simulink model "TrajectoryFollowDemo"  (Simulink 8.2)
settings: Solver=FixedStepDiscrete  StartTime=0.0  StopTime=Inf  RelTol=1e-3
PreLoadFcn:
  | Ts=0.001;
undefined symbols (not defined in the file or in its folder): DiscIntNeverNeededParam
libraries: simulink x8, xpclib x6, speedgoatlib_IO102 x4, speedgoatlib_IO301 x4, xpcutilitieslib x3
settings Model: Creator=LukePH  LastModifiedBy=LukePH  SimulationMode=external  BufferReuse=off
settings DataIOCC: SignalLoggingSaveFormat=Dataset
settings OptimizationCC: BlockReduction=off  OptimizeBlockIOStorage=off  BufferReuse=off  ExpressionFolding=off  ExpressionDepthLimit=128  LocalBlockOutputs=off
settings DebuggingCC: FcnCallInpInsideContextMsg=EnableAllAsError  StateNameClashWarn=none
settings HardwareCC: ProdIntDivRoundTo=Zero  ProdEndianess=LittleEndian  ProdHWDeviceType=Generic->32-bit x86 compatible
settings RTWCC: SystemTargetFile=xpctarget.tlc  TemplateMakefile=xpc_default_tmf  Description=xPC Target  ProcessScript=xpctarget_make_rtw_hook  RTWCompilerOptimization=On
settings xpcTargetCC: TargetFcnLib=ansi_tfl_table_tmw.mat  CodeReplacementLibrary=XPC_BLAS  ParMdlRefBuildCompliant=on  ConcurrentExecutionCompliant=on  CombineSignalStateStructs=off  MATLABClassNameForMDSCustomization=xpcAperiodicCustomization  GRTInterface=on  GenerateAllocFcn=off  xPCTaskExecutionProfile=off  xPCRL32EventNumber=5000  xPCLoadParamSetFile=off  xPCConcurrentTasks=off  xPCEnableSFAnimation=off

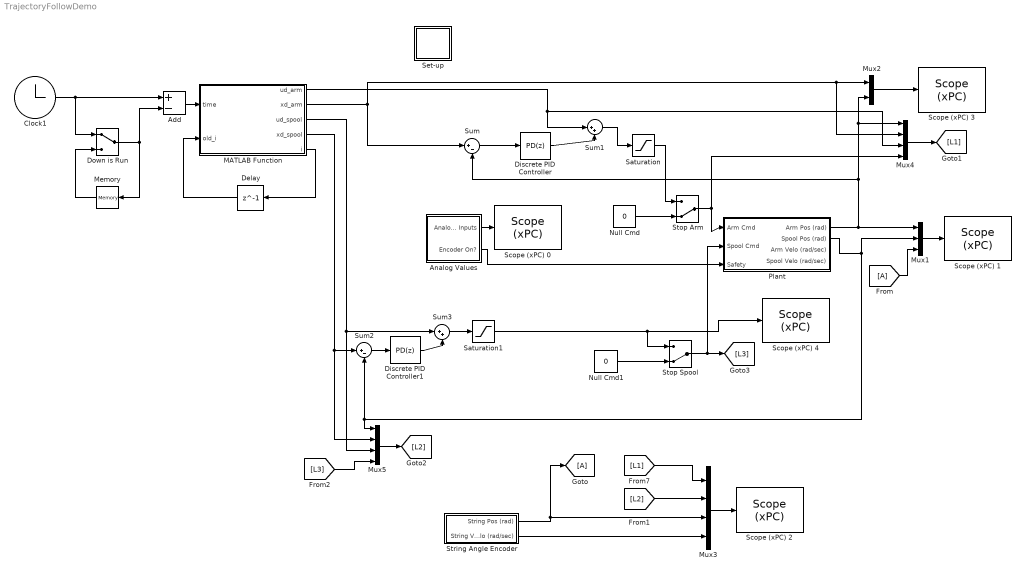
== system TrajectoryFollowDemo ==
  Add : Sum  Inputs=+-
  Analog Values : Subsystem
  Clock1 : Clock
      settings: Decimation=5
  Delay : Delay  DelayLength=1  InitialCondition=1
  Discrete PID Controller : simulink/Continuous/PID Controller  Controller=PD  TimeDomain=Discrete-time  SampleTime=Ts  IntegratorMethod=Forward Euler  FilterMethod=Forward Euler  Form=Parallel  P=30  I=0  D=.15  N=100  InitialConditionSource=internal  InitialConditionForIntegrator=0  InitialConditionForFilter=0  ExternalReset=none  LimitOutput=on  UpperSaturationLimit=6  LowerSaturationLimit=-6  LinearizeAsGain=off  AntiWindupMode=clamping  Kb=1  TrackingMode=off  Kt=1  PParamMin=[]  PParamMax=[]  IParamMin=[]  IParamMax=[]  DParamMin=[]  DParamMax=[]  NParamMin=[]  NParamMax=[]  KbParamMin=[]  KbParamMax=[]  KtParamMin=[]  KtParamMax=[]  POutMin=[]  POutMax=[]  IOutMin=[]  IOutMax=[]  DOutMin=[]  DOutMax=[]  NOutMin=[]  NOutMax=[]  KbOutMin=[]  KbOutMax=[]  KtOutMin=[]  KtOutMax=[]  IntegratorOutMin=[]  IntegratorOutMax=[]  FilterOutMin=[]  FilterOutMax=[]  SumOutMin=[]  SumOutMax=[]  SumI1OutMin=[]  SumI1OutMax=[]  SumI2OutMin=[]  SumI2OutMax=[]  SumI3OutMin=[]  SumI3OutMax=[]  SumDOutMin=[]  SumDOutMax=[]  SaturationOutMin=[]  SaturationOutMax=[]  IntegratorContinuousStateAttributes=''  IntegratorStateMustResolveToSignalObject=off  IntegratorRTWStateStorageClass=Auto  FilterContinuousStateAttributes=''  FilterStateMustResolveToSignalObject=off  FilterRTWStateStorageClass=Auto
  Discrete PID Controller1 : simulink/Continuous/PID Controller  Controller=PD  TimeDomain=Discrete-time  SampleTime=Ts  IntegratorMethod=Forward Euler  FilterMethod=Forward Euler  Form=Parallel  P=20  I=0  D=.05  N=100  InitialConditionSource=internal  InitialConditionForIntegrator=0  InitialConditionForFilter=0  ExternalReset=none  LimitOutput=on  UpperSaturationLimit=6  LowerSaturationLimit=-6  LinearizeAsGain=off  AntiWindupMode=clamping  Kb=1  TrackingMode=off  Kt=1  PParamMin=[]  PParamMax=[]  IParamMin=[]  IParamMax=[]  DParamMin=[]  DParamMax=[]  NParamMin=[]  NParamMax=[]  KbParamMin=[]  KbParamMax=[]  KtParamMin=[]  KtParamMax=[]  POutMin=[]  POutMax=[]  IOutMin=[]  IOutMax=[]  DOutMin=[]  DOutMax=[]  NOutMin=[]  NOutMax=[]  KbOutMin=[]  KbOutMax=[]  KtOutMin=[]  KtOutMax=[]  IntegratorOutMin=[]  IntegratorOutMax=[]  FilterOutMin=[]  FilterOutMax=[]  SumOutMin=[]  SumOutMax=[]  SumI1OutMin=[]  SumI1OutMax=[]  SumI2OutMin=[]  SumI2OutMax=[]  SumI3OutMin=[]  SumI3OutMax=[]  SumDOutMin=[]  SumDOutMax=[]  SaturationOutMin=[]  SaturationOutMax=[]  IntegratorContinuousStateAttributes=''  IntegratorStateMustResolveToSignalObject=off  IntegratorRTWStateStorageClass=Auto  FilterContinuousStateAttributes=''  FilterStateMustResolveToSignalObject=off  FilterRTWStateStorageClass=Auto
  Down is Run : ManualSwitch
  MATLAB Function : MATLAB Function  TreatAsAtomicUnit=on
  Memory : Memory  InheritSampleTime=on
  Mux1 : Mux  Inputs=3
  Mux2 : Mux  Inputs=2
  Mux3 : Mux
  Mux4 : Mux
  Mux5 : Mux
  Null Cmd : Constant  Value=0
  Null Cmd1 : Constant  Value=0
  Plant : Subsystem
  Saturation : Saturate  UpperLimit=6  LowerLimit=-6
  Saturation1 : Saturate  UpperLimit=6  LowerLimit=-6
  "Scope (xPC) 0 " : xpclib/Misc./Scope (xPC)   scopeno=5  scopetype=Target  autostart=on  viewmode=Numerical  formatstr='%15.6f'  grid=on  ylimits=[0,0]  nosamples=250  noprepostsamples=0  interleave=1  triggermode=FreeRun  triggersignal=1  trigsignalfromport=off  triggerlevel=0.0  triggerslope=Either  triggerscope=1  triggersample=0  filename=data.dat  mode=Lazy  writesize=512  autorestart=off  dynamicfilemode=off  maxwritefilesize=512*1024^2
  Scope (xPC) 1 : xpclib/Misc./Scope (xPC)   scopeno=1  scopetype=Target  autostart=on  viewmode=Numerical  formatstr='%15.6f'  grid=on  ylimits=[-2*pi,2*pi]  nosamples=250  noprepostsamples=0  interleave=1  triggermode=FreeRun  triggersignal=1  trigsignalfromport=off  triggerlevel=0.0  triggerslope=Either  triggerscope=1  triggersample=0  filename=data.dat  mode=Lazy  writesize=512  autorestart=off  dynamicfilemode=off  maxwritefilesize=512*1024^2
  Scope (xPC) 2 : xpclib/Misc./Scope (xPC)   scopeno=10  scopetype=File  autostart=on  viewmode=Numerical  formatstr='%15.6f'  grid=on  ylimits=[-2*pi,2*pi]  nosamples=4001  noprepostsamples=0  interleave=4  triggermode=FreeRun  triggersignal=1  trigsignalfromport=off  triggerlevel=0.0  triggerslope=Either  triggerscope=1  triggersample=0  filename=data.dat  mode=Lazy  writesize=512  autorestart=on  dynamicfilemode=off  maxwritefilesize=512*1024^2
  Scope (xPC) 3 : xpclib/Misc./Scope (xPC)   scopeno=6  scopetype=Target  autostart=on  viewmode=Graphical redraw  formatstr='%15.6f'  grid=on  ylimits=[-2*pi,2*pi]  nosamples=250  noprepostsamples=0  interleave=1  triggermode=FreeRun  triggersignal=1  trigsignalfromport=off  triggerlevel=0.0  triggerslope=Either  triggerscope=1  triggersample=0  filename=data.dat  mode=Lazy  writesize=512  autorestart=off  dynamicfilemode=off  maxwritefilesize=512*1024^2
  Scope (xPC) 4 : xpclib/Misc./Scope (xPC)   scopeno=3  scopetype=Target  autostart=on  viewmode=Graphical redraw  formatstr='%15.6f'  grid=on  ylimits=[-2*pi,2*pi]  nosamples=250  noprepostsamples=0  interleave=1  triggermode=FreeRun  triggersignal=1  trigsignalfromport=off  triggerlevel=0.0  triggerslope=Either  triggerscope=1  triggersample=0  filename=data.dat  mode=Lazy  writesize=512  autorestart=off  dynamicfilemode=off  maxwritefilesize=512*1024^2
  Set-up : Subsystem
  Stop Arm : ManualSwitch  CurrentSetting=0
  Stop Spool : ManualSwitch  CurrentSetting=0
  String Angle Encoder : Subsystem
  Sum : Sum  Inputs=|+-
  Sum1 : Sum  Inputs=|++
  Sum2 : Sum  Inputs=|+-
  Sum3 : Sum  Inputs=|++
  wires:
  Delay/1 -> MATLAB Function/2(old_i)
  MATLAB Function/5(i) -> Delay/1
  Clock1/1 -> Add/1, Down is Run/1
  Down is Run/1 -> Memory/1, Add/2
  Memory/1 -> Down is Run/2
  Add/1 -> MATLAB Function/1(time)
  Mux2/1 -> Scope (xPC) 3/1
  Analog Values/1(Analog Inputs) -> "Scope (xPC) 0 "/1
  Plant/1(Arm Pos (rad)) -> Mux1/1, Sum/2, Mux2/2, Mux4/1
  Plant/2(Spool Pos (rad)) -> Mux5/1, Sum2/2, Mux1/2
  Analog Values/2(Encoder On?) -> Plant/3(Safety)
  Sum/1 -> Discrete PID Controller/1
  Null Cmd/1 -> Stop Arm/2
  Saturation/1 -> Stop Arm/1
  Stop Arm/1 -> Plant/1(Arm Cmd), Mux4/4
  Stop Spool/1 -> Plant/2(Spool Cmd), [L3]
  Null Cmd1/1 -> Stop Spool/2
  [A] -> Mux1/3
  Mux1/1 -> Scope (xPC) 1/1
  MATLAB Function/2(xd_arm) -> Sum/1, Mux4/2, Mux2/1
  Mux3/1 -> Scope (xPC) 2/1
  String Angle Encoder/1(String Pos (rad)) -> Mux3/3, [A]
  [L2] -> Mux3/2
  [L1] -> Mux3/1
  Discrete PID Controller/1 -> Sum1/2
  Sum1/1 -> Saturation/1
  Sum2/1 -> Discrete PID Controller1/1
  Discrete PID Controller1/1 -> Sum3/2
  Sum3/1 -> Saturation1/1
  MATLAB Function/4(xd_spool) -> Mux5/2, Sum2/1
  MATLAB Function/3(ud_spool) -> Mux5/3, Sum3/1
  MATLAB Function/1(ud_arm) -> Mux4/3, Sum1/1
  Mux4/1 -> [L1]
  Mux5/1 -> [L2]
  [L3] -> Mux5/4
  String Angle Encoder/2(String Velo (rad/sec)) -> Mux3/4
  Saturation1/1 -> Scope (xPC) 4/1, Stop Spool/1

== system TrajectoryFollowDemo/Analog Values ==
  Analog input : speedgoatlib_IO102/Analog input  id=1  channels=[1,2,3,4]  range=1  high_voltage=off  adCoupling=2  ts=Ts  pciSlot=-1
  Constant : Constant  Value=3.25
  Mux : Mux
  Relational Operator : RelationalOperator  Operator=>  OutDataTypeStr=fixdt(1,16)
  Analog Inputs : Outport
  Encoder On? : Outport  Port=2
  wires:
  Mux/1 -> Analog Inputs/1
  Relational Operator/1 -> Encoder On?/1
  Constant/1 -> Relational Operator/2
  Analog input/1 -> Mux/1
  Analog input/2 -> Mux/2
  Analog input/3 -> Mux/3
  Analog input/4 -> Relational Operator/1, Mux/4

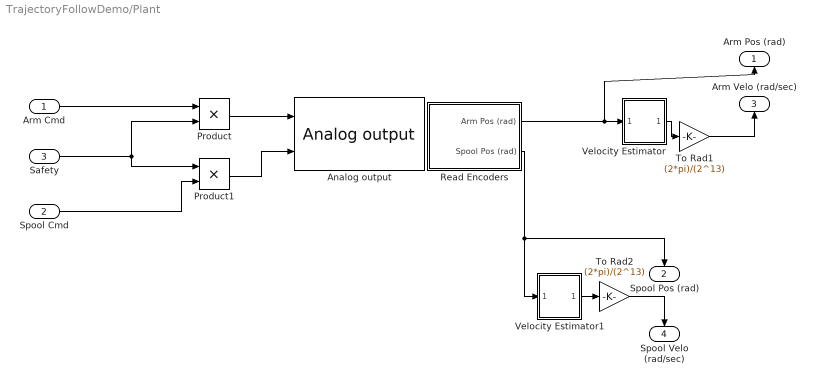
== system TrajectoryFollowDemo/Plant ==
  Arm Cmd : Inport
  Spool Cmd : Inport  Port=2
  Safety : Inport  Port=3
  Analog output : speedgoatlib_IO102/Analog output  id=1  channels=[1,2]  range=1  ts=Ts  pciSlot=-1
  Product : Product
  Product1 : Product
  Read Encoders : Subsystem
  To Rad1 : Gain  Gain=(2*pi)/(2^13)  OutDataTypeStr=double
  To Rad2 : Gain  Gain=(2*pi)/(2^13)  OutDataTypeStr=double
  Velocity Estimator : Subsystem  mask{SampleTime=Ts}
      mask prompts: SampleTime "Sample time (-1 for inherited):"
      mask help:
      | This Block takes in encoder values at a rate of 1 sample per Ts seconds and
      | produces an estimate of the velocity at the given time.
      mask TypeOptions SampleTime: Velocity /SystemSampleTime | Weight Calc/SystemSampleTime | Weighted Average/SystemSampleTime | Velocity /Time Constant/Value | Discrete-Time Integrator/SampleTime | Dead Zone/SampleTime | Weight Calc/9000 rad//sec^2 Cut-off/SampleTime | Weight Calc/Discrete Low Pass1/SampleTime | Weight Calc/Discrete Transfer Fcn/SampleTime | Weight Calc/Discrete Transfer Fcn1/SampleTime | Discrete Low Pass2/SampleTime | Velocity /My Difference/Delay/SampleTime | Velocity /My Difference/Sum/SampleTime
      mask Display:
      | port_label('output', 1, '')
      | port_label('input', 1, '')
  Velocity Estimator1 : Subsystem  mask{SampleTime=Ts}
      mask prompts: SampleTime "Sample time (-1 for inherited):"
      mask help:
      | This Block takes in encoder values at a rate of 1 sample per Ts seconds and
      | produces an estimate of the velocity at the given time.
      mask TypeOptions SampleTime: Velocity /SystemSampleTime | Weight Calc/SystemSampleTime | Weighted Average/SystemSampleTime | Velocity /Time Constant/Value | Discrete-Time Integrator/SampleTime | Dead Zone/SampleTime | Weight Calc/9000 rad//sec^2 Cut-off/SampleTime | Weight Calc/Discrete Low Pass1/SampleTime | Weight Calc/Discrete Transfer Fcn/SampleTime | Weight Calc/Discrete Transfer Fcn1/SampleTime | Discrete Low Pass2/SampleTime | Velocity /My Difference/Delay/SampleTime | Velocity /My Difference/Sum/SampleTime
      mask Display:
      | port_label('output', 1, '')
      | port_label('input', 1, '')
  Arm Pos (rad) : Outport
  Spool Pos (rad) : Outport  Port=2
  Arm Velo (rad/sec) : Outport  Port=3
  Spool Velo (rad/sec) : Outport  Port=4
  wires:
  Read Encoders/2(Spool Pos (rad)) -> Velocity Estimator1/1(In1), Spool Pos (rad)/1
  Spool Cmd/1 -> Product1/2
  Product1/1 -> Analog output/2
  Safety/1 -> Product1/1, Product/2
  Read Encoders/1(Arm Pos (rad)) -> Arm Pos (rad)/1, Velocity Estimator/1(In1)
  Arm Cmd/1 -> Product/1
  Product/1 -> Analog output/1
  Velocity Estimator/1(Out1) -> To Rad1/1
  To Rad1/1 -> Arm Velo (rad/sec)/1
  Velocity Estimator1/1(Out1) -> To Rad2/1
  To Rad2/1 -> Spool Velo (rad/sec)/1

== system TrajectoryFollowDemo/Set-up ==
  AnalogSetUp : Subsystem
  Digital output : speedgoatlib_IO301/DIO/Digital output  id=1  channelGroup=Lower  portType=32 ports of type double  lowerDirection=[0,0,0,0,0,0,1,1,1,1,1,1,1,1,1,1]  upperDirection=[1,1,1,1,1,1,1,1,0,0,0,0,0,0,0,0]  ts=Ts  pciSlot=-1
  Disable NST : Constant  Value=0
  Do Not Zero Arm : Constant
  Do Not Zero Spool : Constant
  Setup : speedgoatlib_IO301/Setup/Setup  group=Lower channel group setup  id=1  fpga1=speedgoat_IO301_CI_01230  pciSlot=-1  lowerDirection=[0,0,0,0,0,0,1,1,1,1,1,1,1,1,1,1]  lowerReset=[1]  lowerValue=[1]  upperDirection=[1, 1, 1, 1, 1, 1, 1, 1, 0, 0, 0, 0, 0, 0, 0, 0]  upperReset=[1]  upperValue=[0]
  wires:
  Disable NST/1 -> Digital output/19, Digital output/17
  Do Not Zero Arm/1 -> Digital output/18
  Do Not Zero Spool/1 -> Digital output/20

== system TrajectoryFollowDemo/String Angle Encoder ==
  EncoderPos3 : xpcutilitieslib/Bit Packing   MaskBitPatterns={[0:12]}  MaskPackDataType=int32  MaskPackDataSize=[1]
  SSIM : speedgoatlib_IO301/SSI/SSIM  id=1  chan=[3]  coding=Binary  clockDivider=[200]  wordSize=[13]  TL=[0]  TP=[990]  ssiminv=off  ts=Ts  pciSlot=-1
  To Rad1 : Gain  Gain=(2*pi)/(2^13)  OutDataTypeStr=double
  To Rad4 : Gain  Gain=(2*pi)/(2^13)  OutDataTypeStr=double
  Velocity Estimator : Subsystem  mask{SampleTime=Ts}
      mask prompts: SampleTime "Sample time (-1 for inherited):"
      mask help:
      | This Block takes in encoder values at a rate of 1 sample per Ts seconds and
      | produces an estimate of the velocity at the given time.
      mask TypeOptions SampleTime: Velocity /SystemSampleTime | Weight Calc/SystemSampleTime | Weighted Average/SystemSampleTime | Velocity /Time Constant/Value | Discrete-Time Integrator/SampleTime | Dead Zone/SampleTime | Weight Calc/9000 rad//sec^2 Cut-off/SampleTime | Weight Calc/Discrete Low Pass1/SampleTime | Weight Calc/Discrete Transfer Fcn/SampleTime | Weight Calc/Discrete Transfer Fcn1/SampleTime | Discrete Low Pass2/SampleTime | Velocity /My Difference/Delay/SampleTime | Velocity /My Difference/Sum/SampleTime
      mask Display:
      | port_label('output', 1, '')
      | port_label('input', 1, '')
  String Pos (rad) : Outport
  String Velo (rad/sec) : Outport  Port=2
  wires:
  To Rad4/1 -> String Pos (rad)/1
  SSIM/1 -> EncoderPos3/1
  EncoderPos3/1 -> Velocity Estimator/1(In1), To Rad4/1
  Velocity Estimator/1(Out1) -> To Rad1/1
  To Rad1/1 -> String Velo (rad/sec)/1

== system TrajectoryFollowDemo/Plant/Read Encoders ==
  EncoderPos : xpcutilitieslib/Bit Packing   MaskBitPatterns={[0:16]}  MaskPackDataType=int32  MaskPackDataSize=[1]
  EncoderPos1 : xpcutilitieslib/Bit Packing   MaskBitPatterns={[0:16]}  MaskPackDataType=int32  MaskPackDataSize=[1]
  SSIM : speedgoatlib_IO301/SSI/SSIM  id=1  chan=[1:2]  coding=Gray  clockDivider=[200]  wordSize=[17]  TL=[0]  TP=[990]  ssiminv=off  ts=Ts  pciSlot=-1
  Spike Removal : Subsystem
  To Rad : Gain  Gain=(2*pi)/(2^17)  OutDataTypeStr=double
  To Rad1 : Gain  Gain=-(2*pi)/(2^17)  OutDataTypeStr=double
  Wrap Encoder Values : Subsystem
  Arm Pos (rad) : Outport
  Spool Pos (rad) : Outport  Port=2
  wires:
  SSIM/1 -> EncoderPos/1
  EncoderPos/1 -> To Rad/1
  To Rad/1 -> Arm Pos (rad)/1
  SSIM/2 -> EncoderPos1/1
  To Rad1/1 -> Spool Pos (rad)/1
  Spike Removal/1(Filtered) -> To Rad1/1
  EncoderPos1/1 -> Wrap Encoder Values/1(Raw Input)
  Wrap Encoder Values/1(Wrapped Values) -> Spike Removal/1(Encoder)

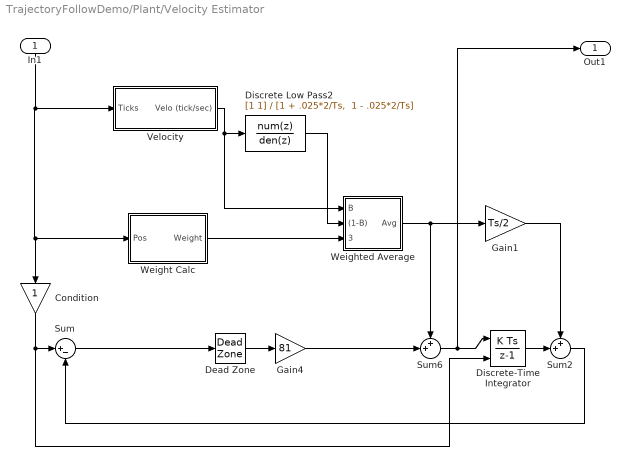
== system TrajectoryFollowDemo/Plant/Velocity Estimator ==
  In1 : Inport
  Condition : Gain  OutMin=0  OutMax=10^9  OutDataTypeStr=double
  Dead Zone : DeadZone  LowerValue=-1  UpperValue=1  SampleTime=SampleTime  SaturateOnIntegerOverflow=on
  Discrete Low Pass2 : DiscreteTransferFcn  Numerator=[1 1]  Denominator="[1 + .025*2/Ts,  1 - .025*2/Ts]"  SampleTime=SampleTime
  Discrete-Time Integrator : DiscreteIntegrator  InitialConditionSource=external  SampleTime=SampleTime  ICPrevOutput=DiscIntNeverNeededParam  ICPrevScaledInput=DiscIntNeverNeededParam
  Gain1 : Gain  Gain=Ts/2
  Gain4 : Gain  Gain=81
  Sum : Sum  Inputs=|+-
  Sum2 : Sum  Inputs=++|
  Sum6 : Sum  Inputs=++|
  "Velocity " : Subsystem  SystemSampleTime=SampleTime
  Weight Calc : Subsystem  SystemSampleTime=SampleTime
  Weighted Average : Subsystem  SystemSampleTime=SampleTime
  Out1 : Outport
  wires:
  Weight Calc/1(Weight) -> Weighted Average/3(Weight)
  Gain1/1 -> Sum2/1
  Discrete-Time Integrator/1 -> Sum2/2
  Sum2/1 -> Sum/2
  Discrete Low Pass2/1 -> Weighted Average/2((1-B))
  Sum6/1 -> Out1/1, Discrete-Time Integrator/1
  Dead Zone/1 -> Gain4/1
  Weighted Average/1(Avg) -> Sum6/1, Gain1/1
  Gain4/1 -> Sum6/2
  Sum/1 -> Dead Zone/1
  "Velocity "/1(Velo (tick/sec)) -> Weighted Average/1("B "), Discrete Low Pass2/1
  In1/1 -> Condition/1, Weight Calc/1(Pos), "Velocity "/1(Ticks)
  Condition/1 -> Discrete-Time Integrator/2, Sum/1

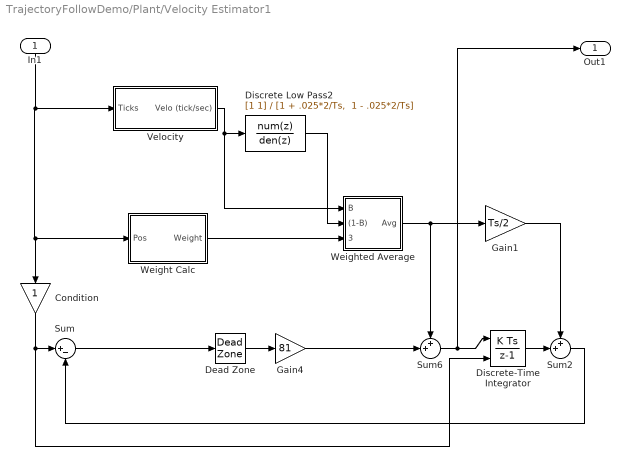
== system TrajectoryFollowDemo/Plant/Velocity Estimator1 ==
  In1 : Inport
  Condition : Gain  OutMin=0  OutMax=10^9  OutDataTypeStr=double
  Dead Zone : DeadZone  LowerValue=-1  UpperValue=1  SampleTime=SampleTime  SaturateOnIntegerOverflow=on
  Discrete Low Pass2 : DiscreteTransferFcn  Numerator=[1 1]  Denominator="[1 + .025*2/Ts,  1 - .025*2/Ts]"  SampleTime=SampleTime
  Discrete-Time Integrator : DiscreteIntegrator  InitialConditionSource=external  SampleTime=SampleTime  ICPrevOutput=DiscIntNeverNeededParam  ICPrevScaledInput=DiscIntNeverNeededParam
  Gain1 : Gain  Gain=Ts/2
  Gain4 : Gain  Gain=81
  Sum : Sum  Inputs=|+-
  Sum2 : Sum  Inputs=++|
  Sum6 : Sum  Inputs=++|
  "Velocity " : Subsystem  SystemSampleTime=SampleTime
  Weight Calc : Subsystem  SystemSampleTime=SampleTime
  Weighted Average : Subsystem  SystemSampleTime=SampleTime
  Out1 : Outport
  wires:
  Weight Calc/1(Weight) -> Weighted Average/3(Weight)
  Gain1/1 -> Sum2/1
  Discrete-Time Integrator/1 -> Sum2/2
  Sum2/1 -> Sum/2
  Discrete Low Pass2/1 -> Weighted Average/2((1-B))
  Sum6/1 -> Out1/1, Discrete-Time Integrator/1
  Dead Zone/1 -> Gain4/1
  Weighted Average/1(Avg) -> Sum6/1, Gain1/1
  Gain4/1 -> Sum6/2
  Sum/1 -> Dead Zone/1
  "Velocity "/1(Velo (tick/sec)) -> Weighted Average/1("B "), Discrete Low Pass2/1
  In1/1 -> Condition/1, Weight Calc/1(Pos), "Velocity "/1(Ticks)
  Condition/1 -> Discrete-Time Integrator/2, Sum/1

== system TrajectoryFollowDemo/Set-up/AnalogSetUp ==
  Analog input : speedgoatlib_IO102/Analog input  Commented=on  id=1  channels=[1,2]  range=1  high_voltage=off  adCoupling=1  ts=Ts  pciSlot=-1
  Mux : Mux  Commented=on  Inputs=2
  Scope (xPC) 1 : xpclib/Misc./Scope (xPC)   Commented=on  scopeno=4  scopetype=Target  autostart=on  viewmode=Graphical redraw  formatstr='%15.6f'  grid=on  ylimits=[0,0]  nosamples=250  noprepostsamples=0  interleave=1  triggermode=FreeRun  triggersignal=1  trigsignalfromport=off  triggerlevel=0.0  triggerslope=Either  triggerscope=1  triggersample=0  filename=data.dat  mode=Lazy  writesize=512  autorestart=off  dynamicfilemode=off  maxwritefilesize=512*1024^2
  SetupAnalog : speedgoatlib_IO102/Setup  group=Analog input setup  id=1  range=+-10V  cal=off  pciSlot=-1  adChannelMode=Multiple-channel (enter number of channels below)  adChannel=4  adCoupling=Single-ended  daChannel=[1,2]  daReset=[1,1]  daInitValue=[0,0]  diChannel=[1]  doChannel=[1]  doReset=[1]  doInitValue=[0]
  wires:
  Mux/1 -> Scope (xPC) 1/1
  Analog input/1 -> Mux/1
  Analog input/2 -> Mux/2

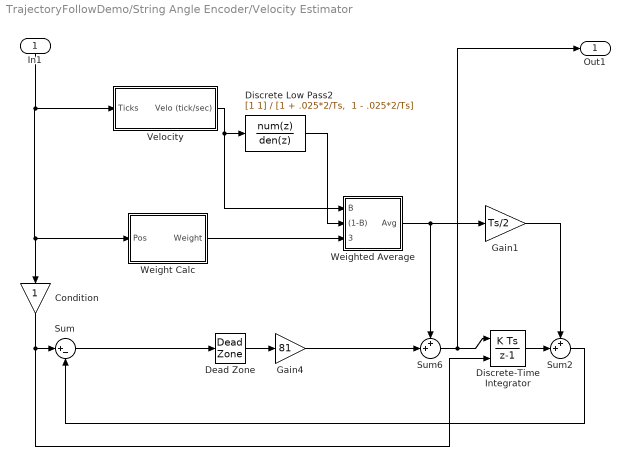
== system TrajectoryFollowDemo/String Angle Encoder/Velocity Estimator ==
  In1 : Inport
  Condition : Gain  OutMin=0  OutMax=10^9  OutDataTypeStr=double
  Dead Zone : DeadZone  LowerValue=-1  UpperValue=1  SampleTime=SampleTime  SaturateOnIntegerOverflow=on
  Discrete Low Pass2 : DiscreteTransferFcn  Numerator=[1 1]  Denominator="[1 + .025*2/Ts,  1 - .025*2/Ts]"  SampleTime=SampleTime
  Discrete-Time Integrator : DiscreteIntegrator  InitialConditionSource=external  SampleTime=SampleTime  ICPrevOutput=DiscIntNeverNeededParam  ICPrevScaledInput=DiscIntNeverNeededParam
  Gain1 : Gain  Gain=Ts/2
  Gain4 : Gain  Gain=81
  Sum : Sum  Inputs=|+-
  Sum2 : Sum  Inputs=++|
  Sum6 : Sum  Inputs=++|
  "Velocity " : Subsystem  SystemSampleTime=SampleTime
  Weight Calc : Subsystem  SystemSampleTime=SampleTime
  Weighted Average : Subsystem  SystemSampleTime=SampleTime
  Out1 : Outport
  wires:
  Weight Calc/1(Weight) -> Weighted Average/3(Weight)
  Gain1/1 -> Sum2/1
  Discrete-Time Integrator/1 -> Sum2/2
  Sum2/1 -> Sum/2
  Discrete Low Pass2/1 -> Weighted Average/2((1-B))
  Sum6/1 -> Out1/1, Discrete-Time Integrator/1
  Dead Zone/1 -> Gain4/1
  Weighted Average/1(Avg) -> Sum6/1, Gain1/1
  Gain4/1 -> Sum6/2
  Sum/1 -> Dead Zone/1
  "Velocity "/1(Velo (tick/sec)) -> Weighted Average/1("B "), Discrete Low Pass2/1
  In1/1 -> Condition/1, Weight Calc/1(Pos), "Velocity "/1(Ticks)
  Condition/1 -> Discrete-Time Integrator/2, Sum/1

== system TrajectoryFollowDemo/Plant/Read Encoders/Spike Removal ==
  Encoder : Inport
  Abs1 : Abs
  Delay1 : Delay  DelayLength=1  InitialCondition=0  SampleTime=Ts
  Memory1 : Memory  InheritSampleTime=on
  Relational Operator2 : RelationalOperator  OutDataTypeStr=boolean
  Spike height : Constant  Value=130000
  Sum2 : Sum  Inputs=|-+
  Switch2 : Switch  Criteria=u2 > Threshold  SampleTime=Ts
  Filtered : Outport
  wires:
  Switch2/1 -> Filtered/1, Memory1/1
  Delay1/1 -> Sum2/1
  Memory1/1 -> Switch2/1
  Encoder/1 -> Sum2/2, Switch2/3, Delay1/1
  Abs1/1 -> Relational Operator2/1
  Spike height/1 -> Relational Operator2/2
  Sum2/1 -> Abs1/1
  Relational Operator2/1 -> Switch2/2

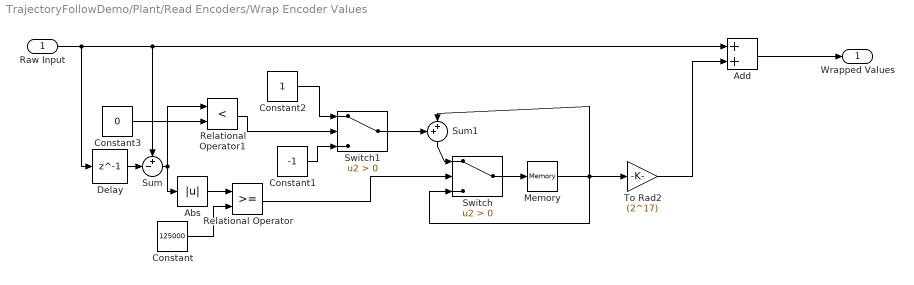
== system TrajectoryFollowDemo/Plant/Read Encoders/Wrap Encoder Values ==
  Raw Input : Inport
  Abs : Abs
  Add : Sum
  Constant : Constant  Value=125000
  Constant1 : Constant  Value=-1
  Constant2 : Constant
  Constant3 : Constant  Value=0
  Delay : Delay  DelayLength=1  InitialCondition=0  SampleTime=Ts
  Memory : Memory  InheritSampleTime=on
  Relational Operator : RelationalOperator  OutDataTypeStr=boolean
  Relational Operator1 : RelationalOperator  Operator=<  OutDataTypeStr=boolean
  Sum : Sum  Inputs=+-|
  Sum1 : Sum  Inputs=++|
  Switch : Switch  Criteria=u2 > Threshold  SampleTime=Ts
  Switch1 : Switch  Criteria=u2 > Threshold  SampleTime=Ts
  To Rad2 : Gain  Gain=(2^17)  OutDataTypeStr=double
  Wrapped Values : Outport
  wires:
  Raw Input/1 -> Delay/1, Sum/1, Add/1
  Add/1 -> Wrapped Values/1
  Constant/1 -> Relational Operator/2
  Relational Operator/1 -> Switch/2
  Sum1/1 -> Switch/1
  Delay/1 -> Sum/2
  Switch/1 -> Memory/1
  Memory/1 -> Sum1/2, Switch/3, To Rad2/1
  Switch1/1 -> Sum1/1
  Constant1/1 -> Switch1/3
  Relational Operator1/1 -> Switch1/2
  Constant2/1 -> Switch1/1
  Sum/1 -> Relational Operator1/1, Abs/1
  Abs/1 -> Relational Operator/1
  Constant3/1 -> Relational Operator1/2
  To Rad2/1 -> Add/2

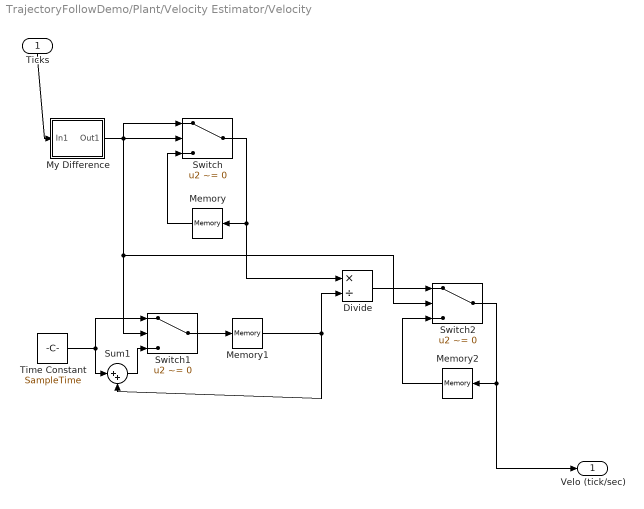
== system TrajectoryFollowDemo/Plant/Velocity Estimator/Velocity  ==
  Ticks : Inport  SampleTime=Ts
  Divide : Product  Inputs=*/
  Memory : Memory
  Memory1 : Memory  X0=Ts
  Memory2 : Memory
  My Difference : Subsystem
  Sum1 : Sum  Inputs=|++
  Switch : Switch  Criteria=u2 ~= 0
  Switch1 : Switch  Criteria=u2 ~= 0
  Switch2 : Switch  Criteria=u2 ~= 0
  Time Constant : Constant  Value=SampleTime
  Velo (tick/sec) : Outport  SampleTime=Ts
  wires:
  Ticks/1 -> My Difference/1(In1)
  My Difference/1(Out1) -> Switch/1, Switch1/2, Switch2/2, Switch/2
  Switch/1 -> Divide/1, Memory/1
  Memory/1 -> Switch/3
  Switch1/1 -> Memory1/1
  Time Constant/1 -> Switch1/1, Sum1/1
  Sum1/1 -> Switch1/3
  Memory1/1 -> Sum1/2, Divide/2
  Divide/1 -> Switch2/1
  Memory2/1 -> Switch2/3
  Switch2/1 -> Velo (tick/sec)/1, Memory2/1

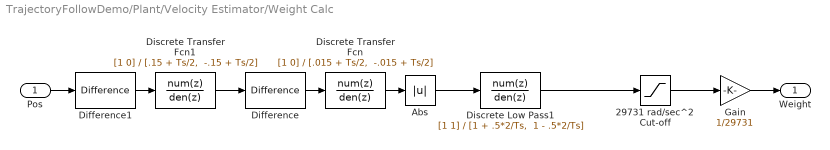
== system TrajectoryFollowDemo/Plant/Velocity Estimator/Weight Calc ==
  Pos : Inport
  29731 rad/sec^2 Cut-off : Saturate  UpperLimit=29731  LowerLimit=0  SampleTime=SampleTime
  Abs : Abs  OutMin=0  OutMax=10^9  OutDataTypeStr=fixdt(1,16)
  Difference : simulink/Discrete/Difference  ICPrevInput=0.0  InputProcessing=Inherited  OutMin=[]  OutMax=[]  OutDataType=fixdt(1, 16)  OutScaling=2^-10  DoSatur=off
  Difference1 : simulink/Discrete/Difference  ICPrevInput=0.0  InputProcessing=Inherited  OutMin=[]  OutMax=[]  OutDataType=fixdt(1, 16)  OutScaling=2^-10  DoSatur=off
  Discrete Low Pass1 : DiscreteTransferFcn  Numerator=[1 1]  Denominator="[1 + .5*2/Ts,  1 - .5*2/Ts]"  SampleTime=SampleTime
  Discrete Transfer Fcn : DiscreteTransferFcn  Numerator=[1 0]  Denominator="[.015 + Ts/2,  -.015 + Ts/2]"  SampleTime=SampleTime
  Discrete Transfer Fcn1 : DiscreteTransferFcn  Numerator=[1 0]  Denominator="[.15 + Ts/2,  -.15 + Ts/2]"  SampleTime=SampleTime
  Gain : Gain  Gain=1/29731
  Weight : Outport  SampleTime=Ts
  wires:
  Gain/1 -> Weight/1
  29731 rad/sec^2 Cut-off/1 -> Gain/1
  Difference1/1 -> Discrete Transfer Fcn1/1
  Difference/1 -> Discrete Transfer Fcn/1
  Discrete Transfer Fcn1/1 -> Difference/1
  Pos/1 -> Difference1/1
  Discrete Transfer Fcn/1 -> Abs/1
  Abs/1 -> Discrete Low Pass1/1
  Discrete Low Pass1/1 -> 29731 rad/sec^2 Cut-off/1

== system TrajectoryFollowDemo/Plant/Velocity Estimator/Weighted Average ==
  "B " : Inport
  (1-B) : Inport  Port=2
  Weight : Inport  Port=3
  Constant : Constant
  Product : Product  RndMeth=Zero
  Product1 : Product  RndMeth=Zero
  Sum : Sum  Inputs=+-|
  Sum1 : Sum  Inputs=++|
  Avg : Outport
  wires:
  "B "/1 -> Product/2
  Weight/1 -> Product/1, Sum/2
  (1-B)/1 -> Product1/2
  Constant/1 -> Sum/1
  Sum/1 -> Product1/1
  Product1/1 -> Sum1/2
  Product/1 -> Sum1/1
  Sum1/1 -> Avg/1

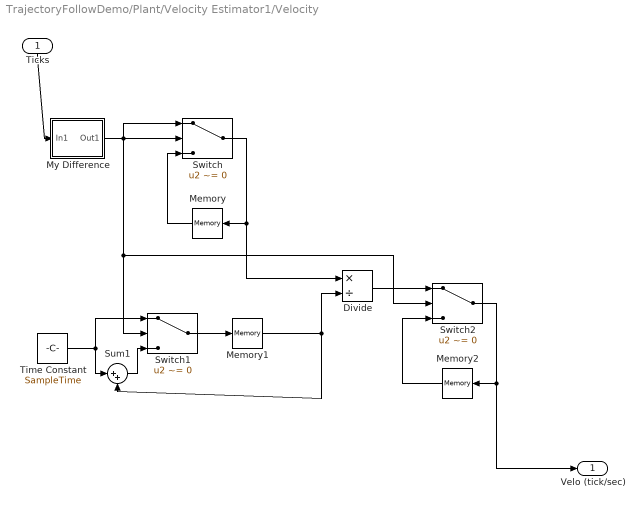
== system TrajectoryFollowDemo/Plant/Velocity Estimator1/Velocity  ==
  Ticks : Inport  SampleTime=Ts
  Divide : Product  Inputs=*/
  Memory : Memory
  Memory1 : Memory  X0=Ts
  Memory2 : Memory
  My Difference : Subsystem
  Sum1 : Sum  Inputs=|++
  Switch : Switch  Criteria=u2 ~= 0
  Switch1 : Switch  Criteria=u2 ~= 0
  Switch2 : Switch  Criteria=u2 ~= 0
  Time Constant : Constant  Value=SampleTime
  Velo (tick/sec) : Outport  SampleTime=Ts
  wires:
  Ticks/1 -> My Difference/1(In1)
  My Difference/1(Out1) -> Switch/1, Switch1/2, Switch2/2, Switch/2
  Switch/1 -> Divide/1, Memory/1
  Memory/1 -> Switch/3
  Switch1/1 -> Memory1/1
  Time Constant/1 -> Switch1/1, Sum1/1
  Sum1/1 -> Switch1/3
  Memory1/1 -> Sum1/2, Divide/2
  Divide/1 -> Switch2/1
  Memory2/1 -> Switch2/3
  Switch2/1 -> Velo (tick/sec)/1, Memory2/1

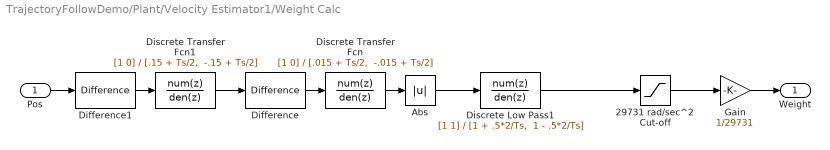
== system TrajectoryFollowDemo/Plant/Velocity Estimator1/Weight Calc ==
  Pos : Inport
  29731 rad/sec^2 Cut-off : Saturate  UpperLimit=29731  LowerLimit=0  SampleTime=SampleTime
  Abs : Abs  OutMin=0  OutMax=10^9  OutDataTypeStr=fixdt(1,16)
  Difference : simulink/Discrete/Difference  ICPrevInput=0.0  InputProcessing=Inherited  OutMin=[]  OutMax=[]  OutDataType=fixdt(1, 16)  OutScaling=2^-10  DoSatur=off
  Difference1 : simulink/Discrete/Difference  ICPrevInput=0.0  InputProcessing=Inherited  OutMin=[]  OutMax=[]  OutDataType=fixdt(1, 16)  OutScaling=2^-10  DoSatur=off
  Discrete Low Pass1 : DiscreteTransferFcn  Numerator=[1 1]  Denominator="[1 + .5*2/Ts,  1 - .5*2/Ts]"  SampleTime=SampleTime
  Discrete Transfer Fcn : DiscreteTransferFcn  Numerator=[1 0]  Denominator="[.015 + Ts/2,  -.015 + Ts/2]"  SampleTime=SampleTime
  Discrete Transfer Fcn1 : DiscreteTransferFcn  Numerator=[1 0]  Denominator="[.15 + Ts/2,  -.15 + Ts/2]"  SampleTime=SampleTime
  Gain : Gain  Gain=1/29731
  Weight : Outport  SampleTime=Ts
  wires:
  Gain/1 -> Weight/1
  29731 rad/sec^2 Cut-off/1 -> Gain/1
  Difference1/1 -> Discrete Transfer Fcn1/1
  Difference/1 -> Discrete Transfer Fcn/1
  Discrete Transfer Fcn1/1 -> Difference/1
  Pos/1 -> Difference1/1
  Discrete Transfer Fcn/1 -> Abs/1
  Abs/1 -> Discrete Low Pass1/1
  Discrete Low Pass1/1 -> 29731 rad/sec^2 Cut-off/1

== system TrajectoryFollowDemo/Plant/Velocity Estimator1/Weighted Average ==
  "B " : Inport
  (1-B) : Inport  Port=2
  Weight : Inport  Port=3
  Constant : Constant
  Product : Product  RndMeth=Zero
  Product1 : Product  RndMeth=Zero
  Sum : Sum  Inputs=+-|
  Sum1 : Sum  Inputs=++|
  Avg : Outport
  wires:
  "B "/1 -> Product/2
  Weight/1 -> Product/1, Sum/2
  (1-B)/1 -> Product1/2
  Constant/1 -> Sum/1
  Sum/1 -> Product1/1
  Product1/1 -> Sum1/2
  Product/1 -> Sum1/1
  Sum1/1 -> Avg/1

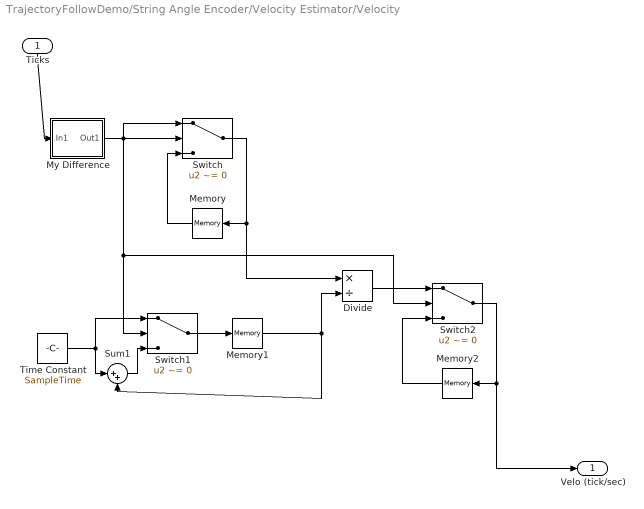
== system TrajectoryFollowDemo/String Angle Encoder/Velocity Estimator/Velocity  ==
  Ticks : Inport  SampleTime=Ts
  Divide : Product  Inputs=*/
  Memory : Memory
  Memory1 : Memory  X0=Ts
  Memory2 : Memory
  My Difference : Subsystem
  Sum1 : Sum  Inputs=|++
  Switch : Switch  Criteria=u2 ~= 0
  Switch1 : Switch  Criteria=u2 ~= 0
  Switch2 : Switch  Criteria=u2 ~= 0
  Time Constant : Constant  Value=SampleTime
  Velo (tick/sec) : Outport  SampleTime=Ts
  wires:
  Ticks/1 -> My Difference/1(In1)
  My Difference/1(Out1) -> Switch/1, Switch1/2, Switch2/2, Switch/2
  Switch/1 -> Divide/1, Memory/1
  Memory/1 -> Switch/3
  Switch1/1 -> Memory1/1
  Time Constant/1 -> Switch1/1, Sum1/1
  Sum1/1 -> Switch1/3
  Memory1/1 -> Sum1/2, Divide/2
  Divide/1 -> Switch2/1
  Memory2/1 -> Switch2/3
  Switch2/1 -> Velo (tick/sec)/1, Memory2/1

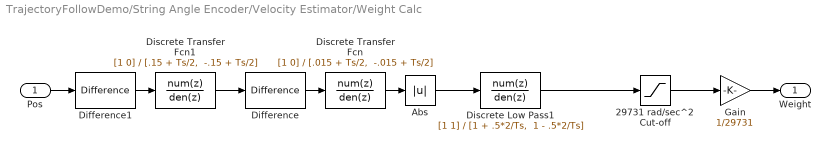
== system TrajectoryFollowDemo/String Angle Encoder/Velocity Estimator/Weight Calc ==
  Pos : Inport
  29731 rad/sec^2 Cut-off : Saturate  UpperLimit=29731  LowerLimit=0  SampleTime=SampleTime
  Abs : Abs  OutMin=0  OutMax=10^9  OutDataTypeStr=fixdt(1,16)
  Difference : simulink/Discrete/Difference  ICPrevInput=0.0  InputProcessing=Inherited  OutMin=[]  OutMax=[]  OutDataType=fixdt(1, 16)  OutScaling=2^-10  DoSatur=off
  Difference1 : simulink/Discrete/Difference  ICPrevInput=0.0  InputProcessing=Inherited  OutMin=[]  OutMax=[]  OutDataType=fixdt(1, 16)  OutScaling=2^-10  DoSatur=off
  Discrete Low Pass1 : DiscreteTransferFcn  Numerator=[1 1]  Denominator="[1 + .5*2/Ts,  1 - .5*2/Ts]"  SampleTime=SampleTime
  Discrete Transfer Fcn : DiscreteTransferFcn  Numerator=[1 0]  Denominator="[.015 + Ts/2,  -.015 + Ts/2]"  SampleTime=SampleTime
  Discrete Transfer Fcn1 : DiscreteTransferFcn  Numerator=[1 0]  Denominator="[.15 + Ts/2,  -.15 + Ts/2]"  SampleTime=SampleTime
  Gain : Gain  Gain=1/29731
  Weight : Outport  SampleTime=Ts
  wires:
  Gain/1 -> Weight/1
  29731 rad/sec^2 Cut-off/1 -> Gain/1
  Difference1/1 -> Discrete Transfer Fcn1/1
  Difference/1 -> Discrete Transfer Fcn/1
  Discrete Transfer Fcn1/1 -> Difference/1
  Pos/1 -> Difference1/1
  Discrete Transfer Fcn/1 -> Abs/1
  Abs/1 -> Discrete Low Pass1/1
  Discrete Low Pass1/1 -> 29731 rad/sec^2 Cut-off/1

== system TrajectoryFollowDemo/String Angle Encoder/Velocity Estimator/Weighted Average ==
  "B " : Inport
  (1-B) : Inport  Port=2
  Weight : Inport  Port=3
  Constant : Constant
  Product : Product  RndMeth=Zero
  Product1 : Product  RndMeth=Zero
  Sum : Sum  Inputs=+-|
  Sum1 : Sum  Inputs=++|
  Avg : Outport
  wires:
  "B "/1 -> Product/2
  Weight/1 -> Product/1, Sum/2
  (1-B)/1 -> Product1/2
  Constant/1 -> Sum/1
  Sum/1 -> Product1/1
  Product1/1 -> Sum1/2
  Product/1 -> Sum1/1
  Sum1/1 -> Avg/1

== system TrajectoryFollowDemo/Plant/Velocity Estimator/Velocity /My Difference ==
  In1 : Inport
  Delay : Delay  DelayLength=1  InitialConditionSource=Input port  SampleTime=Ts
      settings: InputPortMap=u0,p4
  Sum : Sum  Inputs=|+-  SampleTime=Ts
  Out1 : Outport
  wires:
  In1/1 -> Delay/2, Sum/1, Delay/1
  Sum/1 -> Out1/1
  Delay/1 -> Sum/2

== system TrajectoryFollowDemo/Plant/Velocity Estimator1/Velocity /My Difference ==
  In1 : Inport
  Delay : Delay  DelayLength=1  InitialConditionSource=Input port  SampleTime=Ts
      settings: InputPortMap=u0,p4
  Sum : Sum  Inputs=|+-  SampleTime=Ts
  Out1 : Outport
  wires:
  In1/1 -> Delay/2, Sum/1, Delay/1
  Sum/1 -> Out1/1
  Delay/1 -> Sum/2

== system TrajectoryFollowDemo/String Angle Encoder/Velocity Estimator/Velocity /My Difference ==
  In1 : Inport
  Delay : Delay  DelayLength=1  InitialConditionSource=Input port  SampleTime=Ts
      settings: InputPortMap=u0,p4
  Sum : Sum  Inputs=|+-  SampleTime=Ts
  Out1 : Outport
  wires:
  In1/1 -> Delay/2, Sum/1, Delay/1
  Sum/1 -> Out1/1
  Delay/1 -> Sum/2

== matlab function MATLAB Function ==
  data: ud_arm output double; time input double; xd_arm output double; ud_spool output double; xd_spool output double; old_i input double; i output double
function [ud_arm, xd_arm, ud_spool, xd_spool, i] = TrajectoryTimeMap(time,old_i)
%#codegen

% Load Data
D = coder.load('CastingTrajectory.mat');

accu = 10^6;        % Accuracy

if time > max(D.Time) % Check to see if end of simulation
    xd_arm   = D.xd_arm(end);
    ud_arm   = D.ud_arm(end);
    xd_spool = D.xd_spool(end);
    ud_spool = D.ud_spool(end);
    i = old_i;
else % Find closest time
    [Val, I] = min(round(accu*abs(D.Time - time))/accu);
    xd_arm   = D.xd_arm(I);
    ud_arm   = D.ud_arm(I);
    xd_spool = D.xd_spool(I);
    ud_spool = D.ud_spool(I);
    i = I;
end %If
end % Function
